simulink model "Team_4_Project_1_sim_2021a"  (R2021a)
settings: Solver=VariableStepAuto  StartTime=0.0  StopTime=10.0  RelTol=1e-3
undefined symbols (not defined in the file): D, K, mass, small_k
settings Model: Creator=saumilpradhan  LastModifiedBy=saumilpradhan

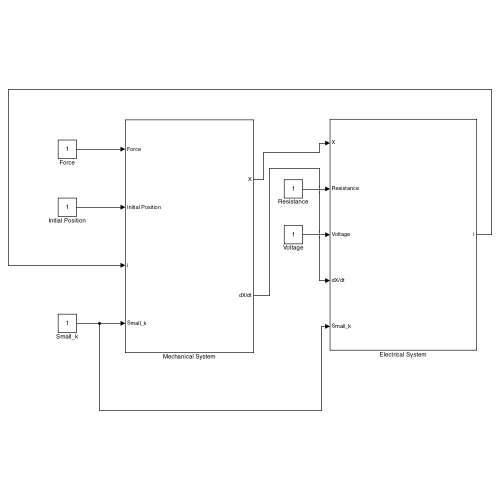
[thumbnail: Simulink's stored preview of the top-level diagram]
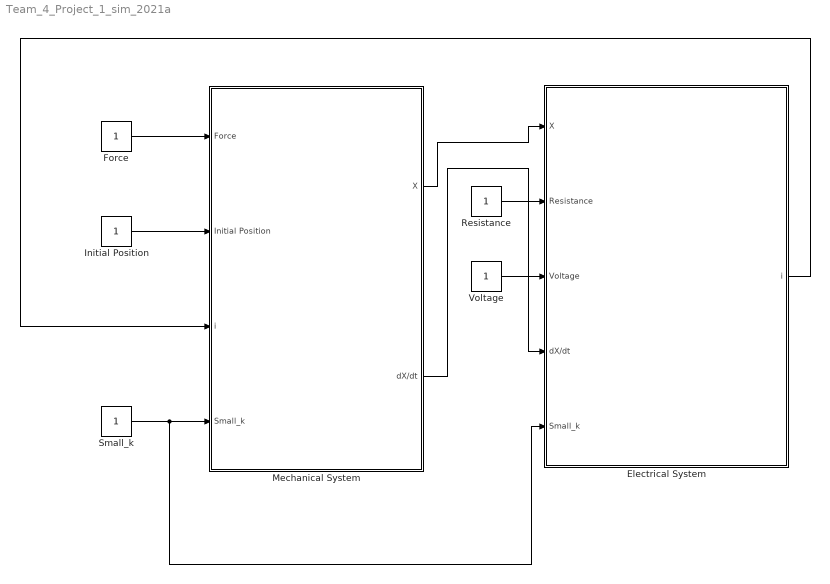
== system Team_4_Project_1_sim_2021a ==
  Electrical System : Subsystem
  Force : Constant
  Initial Position : Constant
  Mechanical System : Subsystem
  Resistance : Constant
  Small_k : Constant
  Voltage : Constant
  wires:
  Mechanical System/2(dX/dt) -> Electrical System/4(dX/dt)
  Voltage/1 -> Electrical System/3(Voltage)
  Force/1 -> Mechanical System/1(Force)
  Electrical System/1(i) -> Mechanical System/3(i)
  Small_k/1 -> Electrical System/5(Small_k), Mechanical System/4(Small_k)
  Resistance/1 -> Electrical System/2(Resistance)
  Mechanical System/1(X) -> Electrical System/1(X)
  Initial Position/1 -> Mechanical System/2(Initial Position)

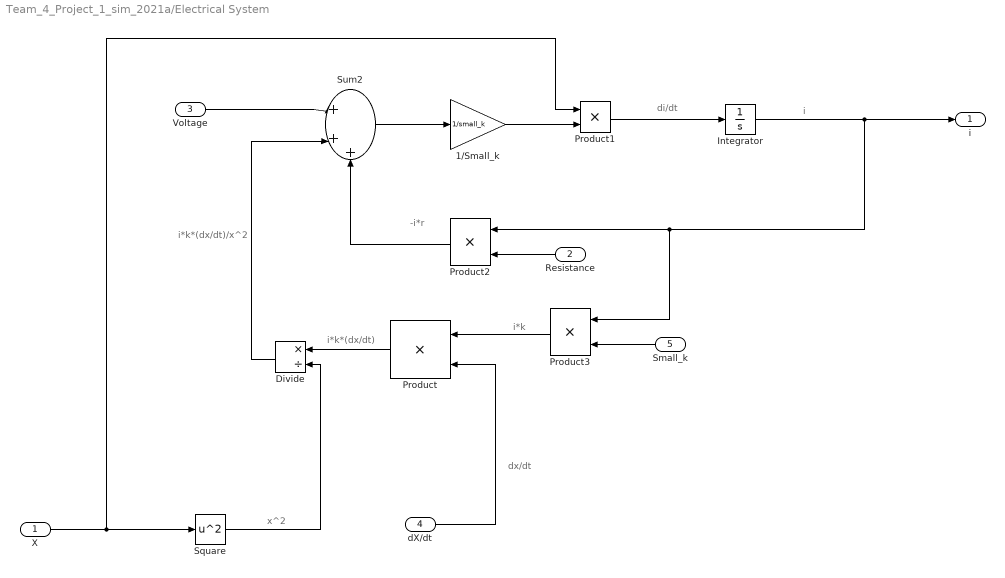
== system Team_4_Project_1_sim_2021a/Electrical System ==
  note: dx/dt
  note: x^2
  note: i
  note: i*k
  note: i*k*(dx/dt)
  note: i*k*(dx/dt)/x^2
  note: -i*r
  note: di/dt
  X : Inport
  Resistance : Inport  Port=2
  Voltage : Inport  Port=3
  dX/dt : Inport  Port=4
  Small_k : Inport  Port=5
  1/Small_k : Gain  Gain=1/small_k
  Divide : Product  Inputs=*/
  Integrator : Integrator
  Product{,1..3} (4 alike) : Product
  Square : Math  Operator=square  SaturateOnIntegerOverflow=on
  Sum2 : Sum  Inputs=|+++
  i : Outport
  wires:
  Product3/1 -> Product/1
  Sum2/1 -> 1/Small_k/1
  dX/dt/1 -> Product/2
  Product/1 -> Divide/1
  Integrator/1 -> i/1, Product3/1, Product2/1
  Voltage/1 -> Sum2/1
  Divide/1 -> Sum2/2
  X/1 -> Product1/1, Square/1
  Square/1 -> Divide/2
  Product1/1 -> Integrator/1
  1/Small_k/1 -> Product1/2
  Product2/1 -> Sum2/3
  Resistance/1 -> Product2/2
  Small_k/1 -> Product3/2

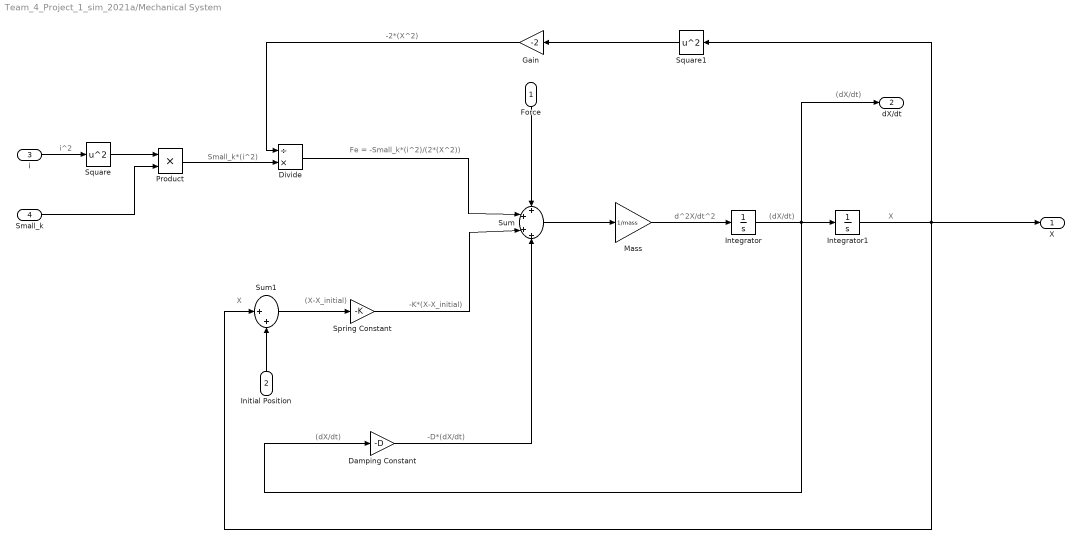
== system Team_4_Project_1_sim_2021a/Mechanical System ==
  note: -D*(dX/dt)
  note: (X-X_initial)
  note: (dX/dt)
  note: -K*(X-X_initial)
  note: d^2X/dt^2
  note: (dX/dt)
  note: X
  note: X
  note: (dX/dt)
  note: i^2
  note: -2*(X^2)
  note: Small_k*(i^2)
  note: Fe = -Small_k*(i^2)/(2*(X^2))
  Force : Inport
  Initial Position : Inport  Port=2
  i : Inport  Port=3
  Small_k : Inport  Port=4
  Damping Constant : Gain  Gain=-D
  Divide : Product  Inputs=/*
  Gain : Gain  Gain=-2
  Integrator : Integrator
  Integrator1 : Integrator
  Mass : Gain  Gain=1/mass
  Product : Product
  Spring Constant : Gain  Gain=-K
  Square : Math  Operator=square  SaturateOnIntegerOverflow=on
  Square1 : Math  Operator=square  SaturateOnIntegerOverflow=on
  Sum : Sum  Inputs=++++
  Sum1 : Sum  Inputs=|++
  X : Outport
  dX/dt : Outport  Port=2
  wires:
  Damping Constant/1 -> Sum/4
  Integrator/1 -> dX/dt/1, Damping Constant/1, Integrator1/1
  Initial Position/1 -> Sum1/2
  Force/1 -> Sum/1
  Integrator1/1 -> Sum1/1, Square1/1, X/1
  Sum1/1 -> Spring Constant/1
  Spring Constant/1 -> Sum/3
  Sum/1 -> Mass/1
  Mass/1 -> Integrator/1
  i/1 -> Square/1
  Square/1 -> Product/1
  Small_k/1 -> Product/2
  Product/1 -> Divide/2
  Square1/1 -> Gain/1
  Gain/1 -> Divide/1
  Divide/1 -> Sum/2
